simulink model "aufgabe_3"  (R2020b)
settings: Solver=VariableStepAuto  StartTime=0.0  StopTime=10.0  RelTol=1e-3
settings Model: Creator=fb3cei  LastModifiedBy=fb3cei

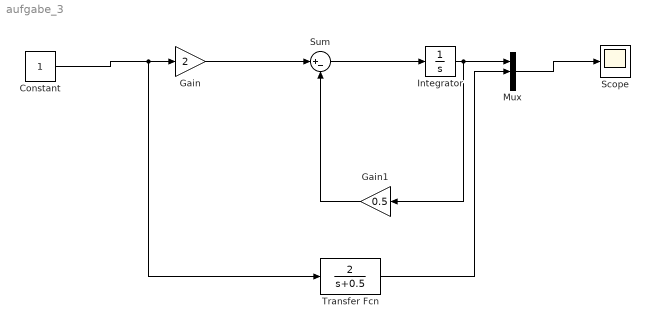
== system aufgabe_3 ==
  Constant : Constant
  Gain : Gain  Gain=2
  Gain1 : Gain  Gain=0.5
  Integrator : Integrator
  Mux : Mux  Inputs=3
  Scope : Scope
  Sum : Sum  Inputs=|+-
  Transfer Fcn : TransferFcn  Numerator=[2]  Denominator=[1 0.5]
  wires:
  Constant/1 -> Transfer Fcn/1, Gain/1
  Gain/1 -> Sum/1
  Sum/1 -> Integrator/1
  Integrator/1 -> Mux/1, Gain1/1
  Mux/1 -> Scope/1
  Gain1/1 -> Sum/2
  Transfer Fcn/1 -> Mux/2
